simulink library "BLE_Library"  (R2017b)
settings: Solver=VariableStepAuto  StartTime=0.0  StopTime=10.0  RelTol=1e-3
values from neighbouring files (symbols this model uses):
  D = D/ScaleCoefficient    [BLE_PostLoad.m]    (also in new_BLE_model.m = zeros(N_BLE,N_BLE+1))
undefined symbols (not defined in the file or in its folder): ADV_IND_AccA, ADV_IND_id, BT_Hop_Separation, BT_Samples_Per_Symbol, CONNECT_IND_id, CONNECT_IND_length, F3B672D172DF, F506B10B1B3E, Header, LL_DATA_EMPTY_length, LL_DATA_id, magnitude, Payload, Preamble, Slot_Ts, T_IFS
libraries: BLE_Library x56, simulink x39, commutil2 x29, dspindex x17, commdigbbndfm2 x5, dspsigops x2, commrandsrc3 x2, dspstat3 x2, dspsrcs4 x1, dsparch4 x1, commdigbbndcpm2 x1
(part 1 of 5)
settings Model: Creator=rolands  LastModifiedBy=rolands

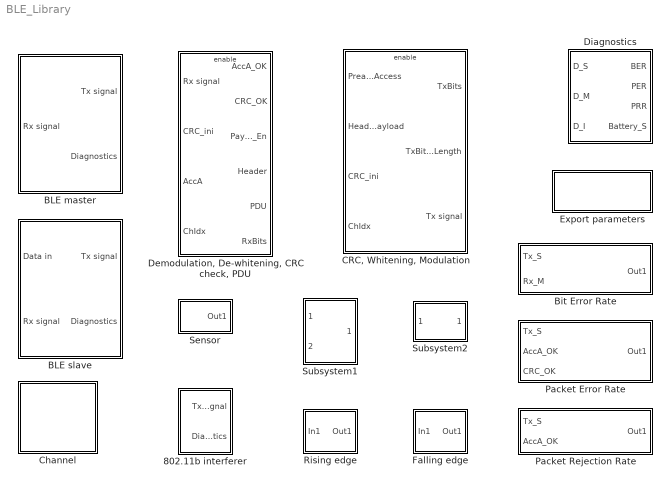
== system BLE_Library ==
  802.11b interferer : Subsystem  mask{rate=70, m=144+48+1024*8 %Preamble + Header + Payload, interference_frequency_number=11}
      mask prompts: rate "Average rate (packets per second):"; m "Mean packet length (us):"; interference_frequency_number "Interference frequency number (1-13, typical: 1, 6 or 11):"
      mask init:
      | interference_frequency_number=min(interference_frequency_number,13);
      | interference_frequency_number=max(interference_frequency_number,1);
      mask Display: disp('802.11b\ninterferer')
  BLE master : Subsystem  StopFcn=|  mask{tON=0, IniState=Initiating, TxAdd=random, InitA_P='112233445566', InitA_R=F506B10B1B3E, PDU_Type=CONNECT_IND, RFU=0, ChSel=0, scanWindow=3500, scanInterval=4500, T_IFS=T_IFS, Interval=6, WinOffset=1, WinSize=1, Timeout=10, Latency=0, SCA=7, DacqSc=MD bit is used (supports only one slave; sampling rate does not exceed 2.136 kHz), NDM=off, DLvalue=off, DataLength=5}
      | uData=get_param(gcb,'UserData');
      | if ~isempty(uData)
      |    if isfield(uData,'AccA_List')
      |       uData=rmfield(uData,'AccA_List');
      |       set_param(gcb,'UserData',uData)
      |    end
      | end
      mask prompts: tON "Turn ON time (us) (>=0 us):"; IniState "Initial state:"; TxAdd "Initiator's address:"; InitA_P "Enter address (hex format, 12 symbols):"; InitA_R "Random address:"; PDU_Type "PDU type:"; scanWindow "Scan window (us) (<=40.96 s):"; scanInterval "Scan interval (us) (<=40.96 s):"; T_IFS "Inter Frame Space (us):"; Interval "Connection Interval (n*1.25 ms, n=6...3200):"; WinOffset "Transmit Window Offset (m*1.25 ms, m=0...n):"; WinSize "Transmit Window Size (k*1.25 ms, k=1...min(8,n-1)):"; Timeout "Connection Supervision Timeout (u*10 ms, u=max(10,floor(n/4)+1)...3200):"; Latency "Connection Slave Latency (0...min(floor(4u/n)-1,499)):"; SCA "Master SCA (0...7):"; NDM "Non-disruptive mode"; DLvalue "Data length is forced to be (1...251 octets):"
      mask init:
      | tON=max(round(tON),0); %minimum value 0 us
      | 
      | scanInterval=min(scanInterval,40.96e6);
      | scanWindow=min(scanWindow,scanInterval);
      | 
      | Interval=max(Interval,6);
      | Interval=min(Interval,3200);
      | 
      | Nsl=ceil(Interval*1250/2500); %max number of slaves in multiple slaves mode
      | 
      | WinOffset=min(WinOffset,Interval);
      | 
      | WinSize=max(WinSize,1);
      | WinSize=min(WinSize,min(8,Interval-1));
      | 
      | Timeout=max(Timeout,max(10,floor(Interval/4)+1));
      | Timeout=min(Timeout,3200);
      | 
      | Latency=max(Latency,0);
      | Latency=min(Latency,min(floor(4*Timeout/Interval)-1,499));
      | 
      | SCA=max(SCA,0);
      | SCA=min(SCA,7);
      | 
      | 
      | switch get_param(gcb,'DacqSc')    %master mode
      |     case 'MD bit is used (supports only one slave; sampling rate does not exceed 2.136 kHz)'        
      |         set_param([gcb,'/Master mode'],'OverrideUsingVariant','OneSlaveMode')     
      |     otherwise
      |         set_param([gcb,'/Master mode'],'OverrideUsingVariant','MultipleSlavesMode')
      | end
      | 
      | 
      | name=get_param(gcb,'name');
      | if name(5)=='m'
      |     nD=name(11:length(name)); %device number
      | elseif name(5)=='s'
      |     nD=name(10:length(name));
      | else
      |     nD='x';
      | end
      | nD=double(nD);
      | 
      | 
      | if strcmp(get_param(gcb,'TxAdd'),'public')
      |     u2=get_param(gcb,'InitA_P');
      |     InitA=dec2bin(hex2dec(u2(2:end-1)),48);
      | else
      |     u2=get_param(gcb,'InitA_R');
      |     InitA=dec2bin(hex2dec(u2),48);
      | end
      | InitA=reshape(InitA.',1,[])-'0';
      | InitA=InitA';
      | 
      | 
      | 
      | slave_AdvAs=zeros(48,8);
      | slave_Names=zeros(1,8);
      | 
      | Names=find_system(bdroot,'regexp','on','Name','BLE slave');
      | if ~isempty(Names)
      |     for k=1:length(Names)
      |         slave_AdvAs(:,k)=getfield(get_param(Names{k},'UserData'),'bin');
      |         name=get_param(Names{k},'Name');
      |         slave_Names(k)=str2num(name(10:end));
      |     end
      | end
      settings: CopyFcn=|
      | if isempty(who('AdvA_List'))
      |    AdvA_List=[];
      | else
      |    AdvA_List=evalin('base','AdvA_List');
      | end
      | 
      | [RandA_bin,RandA_hex, AdvA_List] = GenStatDevAddr(AdvA_List);
      | set_param(gcb,'UserData',struct('bin',RandA_bin,'hex',RandA_hex));
      | set_param(gcb,'InitA_R',RandA_hex);
      settings: DeleteFcn=|
      | if ~isempty(who('AdvA_List'))
      |    AdvA_List=evalin('base','AdvA_List');
      |    add=get_param(gcb,'UserData');
      |    if ~isempty(add)
      |       for k=1:size(AdvA_List,1)
      |          if strcmp(add.hex,AdvA_List(k,:))
      |             AdvA_List(k,:)=[];
      |             break;
      |          end
      |       end
      |    end
      | end
      settings: UndoDeleteFcn=|
      | if isempty(who('AdvA_List'))
      |    AdvA_List=[];
      | else
      |    AdvA_List=evalin('base','AdvA_List');
      | end
      | 
      | add=get_param(gcb,'UserData');
      | if ~isempty(add)
      |    AdvA_List=[AdvA_List; add.hex];
      |    set_param(gcb,'InitA_R',add.hex);
      | else
      |    [RandA_bin,RandA_hex, AdvA_List] = GenStatDevAddr(AdvA_List);
      |    set_param(gcb,'UserData',struct('bin',RandA_bin,'hex',RandA_hex));
      |    set_param(gcb,'InitA_R',RandA_hex);
      | end
      mask TypeOptions IniState: Initiating
      mask TypeOptions TxAdd: public | random
      mask Callback TxAdd:
      | Names = get_param(gcb,'MaskNames');
      | NamesVis = get_param(gcb,'MaskVisibilities');
      | NamesEn = get_param(gcb,'MaskEnables');
      | NameIdx1 = find(strcmp(Names,'InitA_P'));
      | NameIdx2 = find(strcmp(Names,'InitA_R'));
      | 
      | if strcmp(get_param(gcb,'TxAdd'),'public')
      |     NamesVis{NameIdx1}='on';
      |     NamesVis{NameIdx2}='off';
      |     set_param(gcb,'MaskVisibilities',NamesVis);
      | else
      |     NamesVis{NameIdx1}='off';
      |     NamesVis{NameIdx2}='on';
      |     NamesEn{NameIdx2}='off';
      |     set_param(gcb,'MaskVisibilities',NamesVis);
      |     AdvA_List=evalin('base','AdvA_List');
      |     add=get_param(gcb,'UserData');
      |     if isempty(add)
      |         [RandA_bin,RandA_hex, AdvA_List] = GenStatDevAddr(AdvA_List);
      |         assignin('base','AdvA_List',AdvA_List)
      |         add.bin=RandA_bin;
      |         add.hex=RandA_hex;
      |         set_param(gcb,'UserData',add);
      |     else
      |         flag=0;
      |         for k=1:size(AdvA_List,1)
      |             if strcmp(add.hex,AdvA_List(k,:))
      |                 flag=1;
      |                 break;
      |             end
      |         end
      |         if flag~=1
      |             assignin('base','AdvA_List',[AdvA_List;add.hex]);
      |         end
      |     end
      |     set_param(gcb,'InitA_R',add.hex);
      |     set_param(gcb,'MaskEnables',NamesEn);
      | end
      mask TypeOptions PDU_Type: CONNECT_IND
      mask TypeOptions RFU: 0 | 1
      mask TypeOptions ChSel: 0 | 1
      mask TypeOptions DacqSc: MD bit is used (supports only one slave; sampling rate does not exceed 2.136 kHz) | MD bit is ignored (supports multiple slaves; sampling rates do not exceed 0.133 kHz)
      mask Callback DacqSc:
      | Names = get_param(gcb,'MaskNames');
      | NamesVis = get_param(gcb,'MaskVisibilities');
      | NameIdx = find(strcmp(Names,'NDM'));
      | NameIdx1 = find(strcmp(Names,'DLvalue'));
      | NameIdx2 = find(strcmp(Names,'DataLength'));
      | 
      | if strcmp(get_param(gcb,'DacqSc'),'MD bit is used (supports only one slave; sampling rate does not exceed 2.136 kHz)')
      |     NamesVis{NameIdx}='on';
      |     NamesVis{NameIdx1}='on';
      |     NamesVis{NameIdx2}='on';
      |     set_param([gcb,'/Master mode'],'OverrideUsingVariant','OneSlaveMode')
      | else
      |     NamesVis{NameIdx}='off';
      |     NamesVis{NameIdx1}='off';
      |     NamesVis{NameIdx2}='off';
      |     set_param([gcb,'/Master mode'],'OverrideUsingVariant','MultipleSlavesMode')
      | end
      | 
      | set_param(gcb,'MaskVisibilities',NamesVis)
      mask Callback DLvalue:
      | Names = get_param(gcb,'MaskNames');
      | NamesEn = get_param(gcb,'MaskEnables');
      | NameIdx = find(strcmp(Names,'DataLength'));
      | 
      | if strcmp(get_param(gcb,'DLvalue'),'on')
      |     NamesEn{NameIdx}='on';
      | else
      |     NamesEn{NameIdx}='off';
      | end
      | 
      | set_param(gcb,'MaskEnables',NamesEn)
      mask DialogControl Container6 Prompt: Data acquisition mode
      mask Display:
      | if strcmp(get_param(gcb,'TxAdd'),'public')
      |     add=get_param(gcb,'InitA_P');
      |     disp(['PA: ',add(2:end-1),'\n\n\n\n\n\n\n\n\n\n\n\n'])
      | else
      |     disp(['RA: ',get_param(gcb,'InitA_R'),'\n\n\n\n\n\n\n\n\n\n\n\n'])
      | end
      | plot(0,0,100,100,[35,65,65,60,60,35,35],[10,10,90,90,75,75,10],[40,40,60,60,40],[69,50,50,69,69],[48,55,55,50,50,55,55,48],[18,25,25,30,30,35,35,42],[48,43,48,43,43,44,44,48],[30,35,30,25,25,24,24,28],[48,48],[32,42],[48,48],[18,28],[43,44,44,48],[35,36,36,32],[53,49.5,49.5,49.5,49.5,53],[25,28.5,28.5,21.5,21.5,25],[53,49.5,49.5,49.5,49.5,53],[35,38.5,38.5,31.5,31.5,35])
  BLE slave : Subsystem  mask{tON=1, IniState=Advertising, TxAdd=random, AdvA_P='778899AABBCC', AdvA_R=F3B672D172DF, PDU_Type=ADV_IND, RFU=0, ChSel=0, RxAdd=random, TargA_PR=C4CA1158607C, T_ADV_IND_in=1, advInterval_in=20, MDbit=on, NDM=off, SamplParam=2,000 kHz (500 us), 5, 15, 7.5 ms, Fs=1000/500, n_data=5, m_packets=15, Interval_ms=6, BatU=3.6, BatC=2400, Idle_Power=10, Energy_per_sbit=10, Energy_per_rbit=2, BatChargPower=0}
      mask prompts: tON "Turn ON time: (us) (>=1 us)"; IniState "Initial state:"; TxAdd "Advertiser's address:"; AdvA_P "Enter address (hex format, 12 symbols):"; AdvA_R "Random address:"; PDU_Type "PDU type:"; RxAdd "Target's address:"; TargA_PR "Choose from the list:"; T_ADV_IND_in "Time between two consecutive ADV_IND PDUs (ms) (<=10 ms):"; advInterval_in "advInterval (ms) [20 ms ... 10485759.375ms]:"; MDbit "MD bit is used"; NDM "Non-disruptive mode"; SamplParam "Choose from the following:"; Fs "Sampling frequency (kHz):"; n_data "Data length (1 ... 251 octets):"; m_packets "Data packets per connection interval:"; Interval_ms "Required connection interval (n*1.25 ms, n=6...3200):"; BatU "Voltage (V):"; BatC "Capacity (mAh):"; Idle_Power "Idle state power consumption (uW):"; Energy_per_sbit "Energy spent per bit sent (uJ):"; Energy_per_rbit "Energy spent per bit received (uJ):"; BatChargPower "Battery charging power (W):"
      mask init:
      | tON=max(round(tON),1); %minimum value 1 us
      | 
      | T_ADV_IND=round(T_ADV_IND_in*1000); %us
      | T_ADV_IND=min(T_ADV_IND,10000); %maximum value 10 ms
      | 
      | advInterval=round(advInterval_in/0.625)*0.625; %ms
      | advInterval=max(advInterval,20); %minimum value 20 ms 
      | advInterval=min(advInterval,10485759.375); %maximum value 10485759.375 ms
      | advInterval=advInterval*1000; %us
      | 
      | advInterval=max(T_ADV_IND*3,advInterval);
      | 
      | name=get_param(gcb,'name');
      | if name(5)=='m'
      |     nD=name(11:length(name)); %device number
      | elseif name(5)=='s'
      |     nD=name(10:length(name));
      | else
      |     nD='x';
      | end
      | nD=double(nD);
      | 
      | 
      | if strcmp(get_param(gcb,'TxAdd'),'public')
      |     u2=get_param(gcb,'AdvA_P');
      |     AdvA=dec2bin(hex2dec(u2(2:end-1)),48);
      | else
      |     u2=get_param(gcb,'AdvA_R');
      |     AdvA=dec2bin(hex2dec(u2),48);
      | end
      | AdvA=reshape(AdvA.',1,[])-'0';
      | AdvA=AdvA';
      | 
      | u2=get_param(gcb,'TargA_PR');
      | TargA=dec2bin(hex2dec(u2),48);
      | TargA=reshape(TargA.',1,[])-'0';
      | TargA=TargA';
      | 
      | 
      | 
      | master_AdvAs=zeros(48,8);
      | master_Names=zeros(8,1);
      | 
      | Names=find_system(bdroot,'regexp','on','Name','BLE master');
      | if ~isempty(Names)
      |     for k=1:length(Names)
      |         master_AdvAs(:,k)=getfield(get_param(Names{k},'UserData'),'bin');
      |         name=get_param(Names{k},'Name');
      |         master_Names(k)=str2num(name(11:end));
      |     end
      | end
      settings: CopyFcn=|
      | if isempty(who('AdvA_List'))
      |    AdvA_List=[];
      | else
      |    AdvA_List=evalin('base','AdvA_List');
      | end
      | 
      | [RandA_bin,RandA_hex, AdvA_List] = GenStatDevAddr(AdvA_List);
      | set_param(gcb,'UserData',struct('bin',RandA_bin,'hex',RandA_hex));
      | set_param(gcb,'AdvA_R',RandA_hex);
      settings: DeleteFcn=|
      | if ~isempty(who('AdvA_List'))
      |    AdvA_List=evalin('base','AdvA_List');
      |    add=get_param(gcb,'UserData');
      |    if ~isempty(add)
      |       for k=1:size(AdvA_List,1)
      |          if strcmp(add.hex,AdvA_List(k,:))
      |             AdvA_List(k,:)=[];
      |             break;
      |          end
      |       end
      |    end
      | end
      settings: UndoDeleteFcn=|
      | if isempty(who('AdvA_List'))
      |    AdvA_List=[];
      | else
      |    AdvA_List=evalin('base','AdvA_List');
      | end
      | 
      | add=get_param(gcb,'UserData');
      | if ~isempty(add)
      |    AdvA_List=[AdvA_List; add.hex];
      |    set_param(gcb,'AdvA_R',add.hex);
      | else
      |    [RandA_bin,RandA_hex, AdvA_List] = GenStatDevAddr(AdvA_List);
      |    set_param(gcb,'UserData',struct('bin',RandA_bin,'hex',RandA_hex));
      |    set_param(gcb,'AdvA_R',RandA_hex);
      | end
      mask TypeOptions IniState: Advertising
      mask TypeOptions TxAdd: public | random
      mask Callback TxAdd:
      | NamesM = get_param(gcb,'MaskNames');
      | NamesVisM = get_param(gcb,'MaskVisibilities');
      | NamesEnM = get_param(gcb,'MaskEnables');
      | NameMIdx1 = find(strcmp(NamesM,'AdvA_P'));
      | NameMIdx2 = find(strcmp(NamesM,'AdvA_R'));
      | 
      | if strcmp(get_param(gcb,'TxAdd'),'public')
      |     NamesVisM{NameMIdx1}='on';
      |     NamesVisM{NameMIdx2}='off';
      |     set_param(gcb,'MaskVisibilities',NamesVisM);
      | else
      |     NamesVisM{NameMIdx1}='off';
      |     NamesVisM{NameMIdx2}='on';
      |     NamesEnM{NameMIdx2}='off';
      |     set_param(gcb,'MaskVisibilities',NamesVisM);
      |     AdvA_List=evalin('base','AdvA_List');
      |     add=get_param(gcb,'UserData');
      |     if isempty(add)
      |         [RandA_bin,RandA_hex, AdvA_List] = GenStatDevAddr(AdvA_List);
      |         assignin('base','AdvA_List',AdvA_List)
      |         add.bin=RandA_bin;
      |         add.hex=RandA_hex;
      |         set_param(gcb,'UserData',add);
      |     else
      |         flag=0;
      |         for k=1:size(AdvA_List,1)
      |             if strcmp(add.hex,AdvA_List(k,:))
      |                 flag=1;
      |                 break;
      |             end
      |         end
      |         if flag~=1
      |             assignin('base','AdvA_List',[AdvA_List;add.hex]);
      |         end
      |     end
      |     set_param(gcb,'AdvA_R',add.hex);
      |     set_param(gcb,'MaskEnables',NamesEnM);
      | end
      mask TypeOptions PDU_Type: ADV_IND | ADV_DIRECT_IND
      mask Callback PDU_Type:
      | NamesS = get_param(gcb,'MaskNames');
      | NamesVisS = get_param(gcb,'MaskVisibilities');
      | NameSIdx1 = find(strcmp(NamesS,'RxAdd'));
      | NameSIdx2 = find(strcmp(NamesS,'TargA_PR'));
      | hmask=Simulink.Mask.get(gcb);
      | 
      | if strcmp(get_param(gcb,'PDU_Type'),'ADV_IND')
      |     NamesVisS{NameSIdx1}='off';
      |     NamesVisS{NameSIdx2}='off';
      |     hmask.getDialogControl('ConfigureM').Visible='off';
      |     set_param(gcb,'MaskVisibilities',NamesVisS);
      | else
      |     m_Add=[]; kk=1;
      |     Names=find_system(bdroot,'regexp','on','Name','BLE master');
      |     if ~isempty(Names)
      |         for k=1:length(Names)
      |             if strcmp(get_param(Names{k},'TxAdd'),'random')
      |                 addr=get_param(Names{k},'InitA_R');
      |             else
      |                 addr=get_param(Names{k},'InitA_P');
      |                 addr=addr(2:end-1);
      |             end
      |             m_Add=[m_Add; {addr}];
      |             if strcmp(hmask.Parameters(10).Value, addr)
      |                 kk=k;
      |             end
      |         end
      |         hmask.Parameters(10).set('TypeOptions',m_Add,'Value',m_Add{kk});
      |     end
      |     NamesVisS{NameSIdx1}='on';
      |     NamesVisS{NameSIdx2}='on';
      |     hmask.getDialogControl('ConfigureM').Visible='on';
      |     set_param(gcb,'MaskVisibilities',NamesVisS);
      |     set_param(gcb,'RxAdd',get_param(Names{kk},'TxAdd'));
      | end
      mask TypeOptions RFU: 0 | 1
      mask TypeOptions ChSel: 0 | 1
      mask TypeOptions RxAdd: public | random
      mask TypeOptions TargA_PR: C4CA1158607C
      mask Callback TargA_PR:
      | if strcmp(get_param(gcb,'PDU_Type'),'ADV_DIRECT_IND')
      | 
      |     name=get_param(gcb,'TargA_PR');
      |     Names=find_system(bdroot,'regexp','on','Name','BLE master');
      |     if ~isempty(Names)
      |         for k=1:length(Names)
      | 
      |             if strcmp(get_param(Names{k},'TxAdd'),'random')
      |                 initA=get_param(Names{k},'InitA_R');
      |             else
      |                 addr=get_param(Names{k},'InitA_P');
      |                 initA=addr(2:end-1);
      |             end
      | 
      |             if strcmp(name,initA)
      |                 set_param(gcb,'RxAdd',get_param(Names{k},'TxAdd'));
      |                 break;
      |             end
      |         end
      |     end
      | end
      mask Callback MDbit:
      | NamesS = get_param(gcb,'MaskNames');
      | NamesVisS = get_param(gcb,'MaskVisibilities');
      | NamesEnS = get_param(gcb,'MaskEnables');
      | NameSIdx = find(strcmp(NamesS,'NDM'));
      | NameSIdx1 = find(strcmp(NamesS,'SamplParam'));
      | NameSIdx2 = find(strcmp(NamesS,'n_data'));
      | NameSIdx3 = find(strcmp(NamesS,'Interval_ms'));
      | 
      | if strcmp(get_param(gcb,'MDbit'),'on')
      |     NamesVisS{NameSIdx}='on';
      |     NamesVisS{NameSIdx1}='on';
      |     NamesEnS{NameSIdx2}='off';
      |     NamesEnS{NameSIdx3}='off';
      | else
      |     NamesVisS{NameSIdx}='off';
      |     NamesVisS{NameSIdx1}='off';
      |     NamesEnS{NameSIdx2}='on';
      |     NamesEnS{NameSIdx3}='on';
      | end
      | set_param(gcb,'MaskVisibilities',NamesVisS)
      | set_param(gcb,'MaskEnables',NamesEnS)
      | 
      | 
      | if strcmp(get_param(gcb,'MDbit'),'on')
      |     if strcmp(get_param(gcb,'SamplParam'),'2.137 kHz (468 us), 1, 625, 292.5 ms')
      |         set_param(gcb,'Fs','1000/468','n_data','1','m_packets','625','Interval_ms','234');
      |     elseif strcmp(get_param(gcb,'SamplParam'),'2.066 kHz (484 us), 3, 625, 302.5 ms')
      |         set_param(gcb,'Fs','1000/484','n_data','3','m_packets','625','Interval_ms','242');
      |     elseif strcmp(get_param(gcb,'SamplParam'),'2,000 kHz (500 us), 5, 15, 7.5 ms')
      |         set_param(gcb,'Fs','1000/500','n_data','5','m_packets','15','Interval_ms','6');
      |     elseif strcmp(get_param(gcb,'SamplParam'),'1.852 kHz (540 us), 10, 125, 67.5 ms')
      |         set_param(gcb,'Fs','1000/540','n_data','10','m_packets','125','Interval_ms','54');
      |     elseif strcmp(get_param(gcb,'SamplParam'),'1.724 kHz (580 us), 15, 125, 72.5 ms')
      |         set_param(gcb,'Fs','1000/580','n_data','15','m_packets','125','Interval_ms','58');
      |     elseif strcmp(get_param(gcb,'SamplParam'),'1.613 kHz (620 us), 20, 125, 77.5 ms')
      |         set_param(gcb,'Fs','1000/620','n_data','20','m_packets','125','Interval_ms','62');
      |     elseif strcmp(get_param(gcb,'SamplParam'),'1.515 kHz (660 us), 25, 125, 82.5 ms')
      |         set_param(gcb,'Fs','1000/660','n_data','25','m_packets','125','Interval_ms','66');
      |     elseif strcmp(get_param(gcb,'SamplParam'),'1.429 kHz (700 us), 30, 25, 17.5 ms')
      |         set_param(gcb,'Fs','1000/700','n_data','30','m_packets','25','Interval_ms','14');
      |     elseif strcmp(get_param(gcb,'SamplParam'),'1.111 kHz (900 us), 55, 25, 22.5 ms')
      |         set_param(gcb,'Fs','1000/900','n_data','55','m_packets','25','Interval_ms','18');
      |     elseif strcmp(get_param(gcb,'SamplParam'),'0.667 kHz (1500 us), 130, 5, 7.5 ms')
      |         set_param(gcb,'Fs','1000/1500','n_data','130','m_packets','5','Interval_ms','6');
      |     elseif strcmp(get_param(gcb,'SamplParam'),'0.435 kHz (2300 us), 230, 25, 57.5 ms')
      |         set_param(gcb,'Fs','1000/2300','n_data','230','m_packets','25','Interval_ms','46');
      |     else
      |         set_param(gcb,'Fs','1000/7500','n_data','1','m_packets','5','Interval_ms','6');
      |     end
      | else
      |     set_param(gcb,'Fs',['0.8/',get_param(gcb,'Interval_ms'),' (denominator follows from the connection interval)'],'m_packets','1');
      | end
      mask TypeOptions SamplParam: 2.137 kHz (468 us), 1, 625, 292.5 ms | 2.066 kHz (484 us), 3, 625, 302.5 ms | 2,000 kHz (500 us), 5, 15, 7.5 ms | 1.852 kHz (540 us), 10, 125, 67.5 ms | 1.724 kHz (580 us), 15, 125, 72.5 ms | 1.613 kHz (620 us), 20, 125, 77.5 ms | 1.515 kHz (660 us), 25, 125, 82.5 ms | 1.429 kHz (700 us), 30, 25, 17.5 ms | 1.111 kHz (900 us), 55, 25, 22.5 ms | 0.667 kHz (1500 us), 130, 5, 7.5 ms | 0.435 kHz (2300 us), 230, 25, 57.5 ms | 0.133 kHz (7500 us), 1, 5, 7.5 ms (non-uniform)
      mask Callback SamplParam:
      | if strcmp(get_param(gcb,'MDbit'),'on')
      |     if strcmp(get_param(gcb,'SamplParam'),'2.137 kHz (468 us), 1, 625, 292.5 ms')
      |         set_param(gcb,'Fs','1000/468','n_data','1','m_packets','625','Interval_ms','234');
      |     elseif strcmp(get_param(gcb,'SamplParam'),'2.066 kHz (484 us), 3, 625, 302.5 ms')
      |         set_param(gcb,'Fs','1000/484','n_data','3','m_packets','625','Interval_ms','242');
      |     elseif strcmp(get_param(gcb,'SamplParam'),'2,000 kHz (500 us), 5, 15, 7.5 ms')
      |         set_param(gcb,'Fs','1000/500','n_data','5','m_packets','15','Interval_ms','6');
      |     elseif strcmp(get_param(gcb,'SamplParam'),'1.852 kHz (540 us), 10, 125, 67.5 ms')
      |         set_param(gcb,'Fs','1000/540','n_data','10','m_packets','125','Interval_ms','54');
      |     elseif strcmp(get_param(gcb,'SamplParam'),'1.724 kHz (580 us), 15, 125, 72.5 ms')
      |         set_param(gcb,'Fs','1000/580','n_data','15','m_packets','125','Interval_ms','58');
      |     elseif strcmp(get_param(gcb,'SamplParam'),'1.613 kHz (620 us), 20, 125, 77.5 ms')
      |         set_param(gcb,'Fs','1000/620','n_data','20','m_packets','125','Interval_ms','62');
      |     elseif strcmp(get_param(gcb,'SamplParam'),'1.515 kHz (660 us), 25, 125, 82.5 ms')
      |         set_param(gcb,'Fs','1000/660','n_data','25','m_packets','125','Interval_ms','66');
      |     elseif strcmp(get_param(gcb,'SamplParam'),'1.429 kHz (700 us), 30, 25, 17.5 ms')
      |         set_param(gcb,'Fs','1000/700','n_data','30','m_packets','25','Interval_ms','14');
      |     elseif strcmp(get_param(gcb,'SamplParam'),'1.111 kHz (900 us), 55, 25, 22.5 ms')
      |         set_param(gcb,'Fs','1000/900','n_data','55','m_packets','25','Interval_ms','18');
      |     elseif strcmp(get_param(gcb,'SamplParam'),'0.667 kHz (1500 us), 130, 5, 7.5 ms')
      |         set_param(gcb,'Fs','1000/1500','n_data','130','m_packets','5','Interval_ms','6');
      |     elseif strcmp(get_param(gcb,'SamplParam'),'0.435 kHz (2300 us), 230, 25, 57.5 ms')
      |         set_param(gcb,'Fs','1000/2300','n_data','230','m_packets','25','Interval_ms','46');
      |     else
      |         set_param(gcb,'Fs','1000/7500','n_data','1','m_packets','5','Interval_ms','6');
      |     end
      | end
      mask Callback Interval_ms:
      | if strcmp(get_param(gcb,'MDbit'),'off')
      |     set_param(gcb,'Fs',['0.8/',get_param(gcb,'Interval_ms'),' (denominator follows from the connection interval)']);
      | end
      mask DialogControl Container3 Prompt: Sampling parameters
      mask DialogControl ConfigureM Prompt: Configure the master device accordingly
      mask DialogControl ConfigureM Callback:
      | if strcmp(get_param(gcb,'PDU_Type'),'ADV_DIRECT_IND')
      | 
      |     name=get_param(gcb,'TargA_PR');
      |     Names=find_system(bdroot,'regexp','on','Name','BLE master');
      |     if ~isempty(Names)
      |         for k=1:length(Names)
      | 
      |             if strcmp(get_param(Names{k},'TxAdd'),'random')
      |                 initA=get_param(Names{k},'InitA_R');
      |             else
      |                 addr=get_param(Names{k},'InitA_P');
      |                 initA=addr(2:end-1);
      |             end
      | 
      |             if strcmp(name,initA)
      |                 set_param(Names{k},'Interval',get_param(gcb,'Interval_ms'));
      | 
      |                 NamesM = get_param(Names{k},'MaskNames');
      |                 NamesVisM = get_param(Names{k},'MaskVisibilities');
      |                 NameMIdx1 = find(strcmp(NamesM,'NDM'));
      |                 NameMIdx2 = find(strcmp(NamesM,'DLvalue'));
      |                 NameMIdx3 = find(strcmp(NamesM,'DataLength'));
      | 
      |                 if strcmp(get_param(gcb,'MDbit'),'on')
      |                     set_param(Names{k},'DacqSc','MD bit is used (supports only one slave; sampling rate does not exceed 2.136 kHz)')
      |                     set_param([Names{k},'/Master mode'],'OverrideUsingVariant','OneSlaveMode')
      |                     ndm=get_param(gcb,'NDM');
      |                     NamesVisM{NameMIdx1}='on';
      |                     NamesVisM{NameMIdx2}='on';
      |                     NamesVisM{NameMIdx3}='on';
      |                 else
      |                     set_param(Names{k},'DacqSc','MD bit is ignored (supports multiple slaves; sampling rates do not exceed 0.133 kHz)')
      |                     set_param([Names{k},'/Master mode'],'OverrideUsingVariant','MultipleSlavesMode')
      |                     ndm='off';
      |                     NamesVisM{NameMIdx1}='off';
      |                     NamesVisM{NameMIdx2}='off';
      |                     NamesVisM{NameMIdx3}='off';
      |                 end
      | 
      |                 set_param(Names{k},'MaskVisibilities',NamesVisM)
      |                 set_param(Names{k},'NDM',ndm)
      |                 set_param(Names{k},'DataLength',get_param(gcb,'n_data'))
      |                 break;
      |             end
      |         end
      |     end
      | end
      mask DialogControl Container6 Prompt: Battery parameters
      mask Display:
      | if strcmp(get_param(gcb,'TxAdd'),'public')
      |     add=get_param(gcb,'AdvA_P');
      |     disp(['PA: ',add(2:end-1),'\n\n\n\n\n\n\n\n\n\n\n\n'])
      | else
      |     disp(['RA: ',get_param(gcb,'AdvA_R'),'\n\n\n\n\n\n\n\n\n\n\n\n'])
      | end
      | 
      | if strcmp(get_param(gcb,'PDU_Type'),'ADV_DIRECT_IND')
      |     add=get_param(gcb,'TargA_PR');
      |     if strcmp(get_param(gcb,'RxAdd'),'public')
      |         disp(['\n\n\n\n\n\n\n\n\n\n\n\n','TA: ',add(2:end-1)])
      |     else
      |         disp(['\n\n\n\n\n\n\n\n\n\n\n\n','TA: ',add])
      |     end
      | end
      | 
      | plot(0,0,100,100,[35,65,65,60,60,35,35],[10,10,90,90,75,75,10],[40,40,60,60,40],[69,50,50,69,69],[48,55,55,50,50,55,55,48],[18,25,25,30,30,35,35,42],[48,43,48,43,43,44,44,48],[30,35,30,25,25,24,24,28],[48,48],[32,42],[48,48],[18,28],[43,44,44,48],[35,36,36,32],[53,49.5,49.5,49.5,49.5,53],[25,28.5,28.5,21.5,21.5,25],[53,49.5,49.5,49.5,49.5,53],[35,38.5,38.5,31.5,31.5,35])
  Bit Error Rate : Subsystem
      mask Display: disp('BER\n calculation')
  "CRC, Whitening, Modulation" : Subsystem
  Channel : Subsystem  InitFcn=|  mask{Tx_power=0, Channel_SNR=-20, InterfOn=off, Interf_power=10}
      | XY=[];
      | Names=find_system(bdroot,'regexp','on','Name','BLE master');
      | if ~isempty(Names)
      |     for k=1:length(Names)
      |         xy=get_param(Names{k},'Position');
      |         XY=[XY;xy(1:2)];
      |     end
      | end
      | 
      | Names=find_system(bdroot,'regexp','on','Name','BLE slave');
      | if ~isempty(Names)
      |     for k=1:length(Names)
      |         xy=get_param(Names{k},'Position');
      |         XY=[XY;xy(1:2)];
      |     end
      | end
      | 
      | Names=find_system(bdroot,'regexp','on','Name','interferer');
      | if ~isempty(Names)
      |     for k=1:length(Names)
      |         xy=get_param(Names{k},'Position');
      |         XY=[XY;xy(1:2)];
      |     end
      | end
      | 
      | if ~isempty(XY)
      |     N_BLE=size(XY,1)-1;
      |     D=zeros(N_BLE,N_BLE+1);
      |     for n=1:size(XY,1)
      |         for k=1:size(XY,1)
      |             D(n,k)=sqrt((XY(n,1)-XY(k,1))^2+(XY(n,2)-XY(k,2))^2);
      |         end
      |     end
      |     ScaleCoefficient=0;
      |     varList=whos(get_param(bdroot,'ModelWorkspace'));
      |     if ~isempty(varList)
      |         for m=1:length(varList)
      |             if strcmp(varList(m).name,'ScaleCoefficient')
      |                 ScaleCoefficient=getVariable(get_param(bdroot,'ModelWorkspace'),'ScaleCoefficient');
      |                 break;
      |             end
      |         end
      |     end
      |     if ScaleCoefficient==0
      |         ScaleCoefficient=1;
      |     end
      |     D=D/ScaleCoefficient;
      |     
      |     D_path_loss=1./(4*pi*D*2.4e9/299792458);
      |     D_path_loss(D_path_loss==Inf)=0;
      |     assignin('base', 'D', D');
      |     assignin('base', 'D_path_loss_I_on', D_path_loss');
      |     D_path_loss(:,end)=0;
      |     assignin('base', 'D_path_loss_I_off', D_path_loss');
      | end
      mask prompts: Tx_power "BLE transmit power (-20 dBm ... +10 dBm):"; Channel_SNR "AWGN channel noise power (dBm):"; InterfOn "Interferer On"; Interf_power "Interferer transmit power (<= +20 dBm):"
  "Demodulation, De-whitening, CRC check, PDU" : Subsystem  mask{PDU_Length=112 %ADV_DIRECT_IND: 2+6+6 octets (H,AdvA,TargetA), N_after=136 %max PDU length + CRC}
      mask prompts: PDU_Length "PDU length (number of bits):"; N_after "Counter limit after AccA OK:"
  Diagnostics : Subsystem
  Export parameters : Subsystem
      settings: OpenFcn=|
      | if ~exist('Parameters','dir')
      |     mkdir('Parameters')
      | end
      | 
      | set_param(gcb,'BackgroundColor','red')
      | set_param(gcb,'MaskDisplay',"disp('Generating\n.txt file')")
      | pause(0.5)
      | 
      | Names=find_system(bdroot,'regexp','on','Name','BLE master');
      | if ~isempty(Names)
      |     for k=1:length(Names)
      |        ParamNames=get_param(Names{k},'MaskPrompts');
      |        ParamValues=get_param(Names{k},'MaskValues');
      |        writetable(table(ParamNames, ParamValues, 'VariableNames',{'Parameter','Value'}), ['Parameters/Parameters_',get_param(Names{k},'Name'),'.txt'])
      |     end
      | end
      | 
      | Names=find_system(bdroot,'regexp','on','Name','BLE slave');
      | if ~isempty(Names)
      |     for k=1:length(Names)
      |        ParamNames=get_param(Names{k},'MaskPrompts');
      |        ParamValues=get_param(Names{k},'MaskValues');
      |        writetable(table(ParamNames, ParamValues, 'VariableNames',{'Parameter','Value'}), ['Parameters/Parameters_',get_param(Names{k},'Name'),'.txt'])
      |     end
      | end
      | 
      | set_param(gcb,'BackgroundColor','green')
      | set_param(gcb,'MaskDisplay',"disp('Double-click\nto generate\nparameters .txt files')")
      mask Display: disp('Double-click\nto generate\nparameters .txt files')
  Falling edge : Subsystem
      mask Display: disp('Falling\nedge\npulse')
  Packet Error Rate : Subsystem
      mask Display: disp('PER\n calculation')
  Packet Rejection Rate : Subsystem
      mask Display: disp('PRR\n calculation')
  Rising edge : Subsystem
      mask Display: disp('Rising\nedge\npulse')
  Sensor : Subsystem  mask{NbitsPerSample=4}
      mask prompts: NbitsPerSample "Number of bits per sample:"
      mask Display: disp('Sensor')
  Subsystem1 : Subsystem  mask{PDU_type=CONNECT_IND_id}
      mask prompts: PDU_type "PDU type:"
  Subsystem2 : Subsystem  mask{offset=1}
      mask Display: disp('Count\npulses')

== system BLE_Library/802.11b interferer ==
  22MHz white noise : dspsrcs4/Random Source  SrcType=Gaussian  NormMethod=Ziggurat  CltLength=12  MinVal=0  MaxVal=1  MeanVal=0  VarVal=1  RepMode=Not repeatable  rawSeed=awgn_seed  IsInherit=off  SampMode=Discrete  SampTime=Slot_Ts/22  SampFrame=22  DataType=Double  OutComplex=Complex  OutputFrames=off
  Bus Creator : BusCreator  Inputs=2
  Constant1 : Constant  SampleTime=Slot_Ts
  Constant5 : Constant  Value=interference_frequency_number  SampleTime=Slot_Ts
  Digital Filter Design : dsparch4/Digital Filter Design  mwdsp_browser_bugfix_var=off
  Enabled Subsystem : Subsystem  TreatAsAtomicUnit=on
  Gain : Gain  Gain=sqrt(4)  SaturateOnIntegerOverflow=on  OutDataTypeStr=Inherit: Same as input  ParamDataTypeStr=Inherit: Same as input
  Gain1 : Gain  Gain=2.7  SaturateOnIntegerOverflow=on  OutDataTypeStr=Inherit: Same as input  ParamDataTypeStr=Inherit: Same as input
  M-FSK Modulator Baseband : commdigbbndfm2/M-FSK Modulator Baseband  M=13  InType=Integer  Enc=Binary  freqSep=5e6  phaseType=Continuous  numSamp=BT_Samples_Per_Symbol  RateOptions=Enforce single-rate processing  outDataType=double
      settings: SourceProductName=Communications System Toolbox
  Mix to appropriate hop frequency : Product  SaturateOnIntegerOverflow=on  InputSameDT=on  OutDataTypeStr=Inherit: Same as first input
  Poisson pulses : Subsystem  mask{average_rate=rate, packet_length=m*Slot_Ts}
      mask prompts: average_rate "Average rate (packets per second):"; packet_length "Mean packet length:"
      mask init:
      | adjusted_rate=1/(1/average_rate-packet_length);
  Sum : Sum  Inputs=|+-
  Upsample to 88 MHz : dspsigops/Upsample  N=4  phase=0  InputProcessing=Columns as channels (frame based)  RateOptions=Enforce single-rate processing  ic=0  mode=Unused parameter value
  Tx signal : Outport
  Diagnostics : Outport  Port=2
  wires:
  Mix to appropriate hop frequency/1 -> Enabled Subsystem/1(In1)
  Digital Filter Design/1 -> Gain1/1
  Upsample to 88 MHz/1 -> Gain/1
  Gain/1 -> Digital Filter Design/1
  22MHz white noise/1 -> Upsample to 88 MHz/1
  Poisson pulses/1(enable) -> Enabled Subsystem/Enable, Bus Creator/1  "Interf ON"
  M-FSK Modulator Baseband/1 -> Mix to appropriate hop frequency/2
  Constant5/1 -> Sum/1
  Constant1/1 -> Sum/2
  Sum/1 -> Bus Creator/2, M-FSK Modulator Baseband/1  "Interf freq idx"
  Enabled Subsystem/1(Out3) -> Tx signal/1
  Gain1/1 -> Mix to appropriate hop frequency/1
  Bus Creator/1 -> Diagnostics/1

== system BLE_Library/BLE master ==
  Rx signal : Inport
  Constant1 : Constant  SampleTime=Slot_Ts
  Constant4 : Constant  OutDataTypeStr=boolean  SampleTime=Slot_Ts
  Manual Switch1 : ManualSwitch
  Manual Switch4 : ManualSwitch
  Master mode : Subsystem  Variant=on  OverrideUsingVariant=OneSlaveMode
  Rising edge : BLE_Library/Rising edge  SystemSampleTime=-1
  Subsystem7 : Subsystem
      mask Display: disp('Rx\nOn/Off')
  Turn ON time : Delay  DelayLength=tON  InitialCondition=0  SampleTime=Slot_Ts
  Unit Delay1 : UnitDelay  SampleTime=Slot_Ts
  Tx signal : Outport
  Diagnostics : Outport  Port=2
  wires:
  Manual Switch4/1 -> Master mode/3(In3)
  Manual Switch1/1 -> Master mode/2(Rx signal)
  Rising edge/1 -> Master mode/1(Turn ON)
  Master mode/2(Diagnostics) -> Diagnostics/1
  Master mode/1(Tx signal) -> Tx signal/1
  Rx signal/1 -> Unit Delay1/1
  Unit Delay1/1 -> Subsystem7/1(In1), Manual Switch1/1
  Subsystem7/2(Out2) -> Manual Switch4/2
  Constant4/1 -> Manual Switch4/1
  Subsystem7/1(Out1) -> Manual Switch1/2
  Constant1/1 -> Turn ON time/1
  Turn ON time/1 -> Rising edge/1

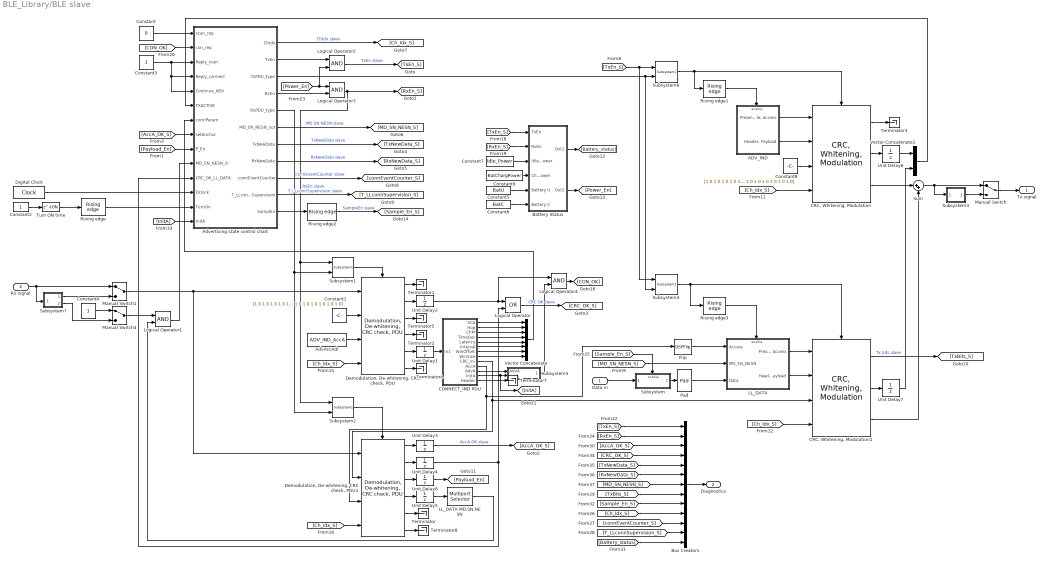
== system BLE_Library/BLE slave ==
  "Data in " : Inport
  Rx signal : Inport  Port=2
  ADV_IND : Subsystem  TreatAsAtomicUnit=on
  AdvAccAdr : Constant  Value=ADV_IND_AccA  VectorParams1D=off  SampleTime=Slot_Ts
  Advertising state control chart : Stateflow chart  TreatAsAtomicUnit=on
  Battery Status : Subsystem
  Bus Creator1 : BusCreator  Inputs=13
  CONNECT_IND PDU : Subsystem
  "CRC, Whitening, Modulation" : BLE_Library/CRC, Whitening,  Modulation
  "CRC, Whitening, Modulation1" : BLE_Library/CRC, Whitening,  Modulation
  Constant : Constant  Value=0  SampleTime=Slot_Ts
  Constant1 : Constant  Value=[1 0 1 0 1 0 1 0 1 0 1 0 1 0 1 0 1 0 1 0 1 0 1 0]  OutDataTypeStr=boolean  SampleTime=Slot_Ts
  Constant2 : Constant  SampleTime=Slot_Ts
  Constant3 : Constant  SampleTime=Slot_Ts
  Constant4 : Constant  OutDataTypeStr=boolean  SampleTime=Slot_Ts
  Constant5 : Constant  Value=BatU  SampleTime=Slot_Ts
  Constant6 : Constant  Value=BatC  SampleTime=Slot_Ts
  Constant7 : Constant  Value=Idle_Power  SampleTime=Slot_Ts
  Constant8 : Constant  Value=[1 0 1 0 1 0 1 0 1 0 1 0 1 0 1 0 1 0 1 0 1 0 1 0]  OutDataTypeStr=boolean  SampleTime=Slot_Ts
  Constant9 : Constant  Value=BatChargPower  SampleTime=Slot_Ts
  "Demodulation, De-whitening, CRC check, PDU" : BLE_Library/Demodulation, De-whitening, CRC check, PDU  PDU_Length=288 %CONNECT_IND: 2+6+6+22 octets (H,InitA,AdvA,LLData)  N_after=312 %max PDU length + CRC
  "Demodulation, De-whitening, CRC check, PDU1" : BLE_Library/Demodulation, De-whitening, CRC check, PDU  PDU_Length=2 %PDU is not required  N_after=40 %max PDU length + CRC
  Digital Clock : DigitalClock  SampleTime=Slot_Ts
  Flip : DSPFlip
  LL_DATA : Subsystem
  LL_DATA MD,SN,NESN : dspindex/Multiport Selector  rowsOrCols=Rows  idxCellArray={12:14}  idxErrMode=Clip Index
  Logical Operator : Logic  Operator=OR  AllPortsSameDT=off  OutDataTypeStr=boolean
  Logical Operator{1..4} (4 alike) : Logic  AllPortsSameDT=off  OutDataTypeStr=boolean
  Manual Switch : ManualSwitch
  Manual Switch1 : ManualSwitch
  Manual Switch4 : ManualSwitch
  Pad : dspsigops/Pad  padAlong=Columns  dimsToPad=1  valSrc=Specify via dialog  padVal=0  spec=Output size  padNumOutRowsSpecMethod=User-specified  numOutRows=n_data*8  padNumOutColsSpecMethod=User-specified  numOutCols=1  isVarDimsMode=off  padBeginning=0  padEnd=0  outSizeMode=User-specified  outSize=1  padSigAt=End  trunc_flag=Warning  roundingMode=Floor  overflowMode=off  truncOrWrapMode=Truncate  wrap_flag=None
      settings: SourceProductName=DSP System Toolbox  SourceProductBaseCode=DS
  Rising edge{,1..3} (4 alike) : BLE_Library/Rising edge  SystemSampleTime=-1
  Subsystem : Subsystem
  Subsystem1 : BLE_Library/Subsystem1  PDU_type=CONNECT_IND_id
  Subsystem2 : BLE_Library/Subsystem1  PDU_type=LL_DATA_id
  Subsystem3 : Subsystem
      mask Display: disp('Tx\nOn/Off')
  Subsystem4 : BLE_Library/Subsystem1  PDU_type=LL_DATA_id
  Subsystem5 : Subsystem
  Subsystem6 : BLE_Library/Subsystem1  PDU_type=ADV_IND_id
  Subsystem7 : Subsystem
      mask Display: disp('Rx\nOn/Off')
  Sum : Sum  Inputs=|++
  Terminator{,1..5,7..8} (8 alike) : Terminator
  Turn ON time : Delay  DelayLength=tON  InitialCondition=0  SampleTime=Slot_Ts
  Unit Delay{1..8} (8 alike) : UnitDelay  SampleTime=Slot_Ts
  Vector Concatenate : Concatenate  NumInputs=8
  Vector Concatenate1 : Concatenate
  Tx signal : Outport
  Diagnostics : Outport  Port=2
  wires:
  Rising edge3/1 -> LL_DATA/Enable
  Subsystem4/1 -> Rising edge3/1, "CRC, Whitening, Modulation1"/Enable
  Rising edge1/1 -> ADV_IND/Enable
  Unit Delay6/1 -> Vector Concatenate1/1
  Subsystem6/1 -> "CRC, Whitening, Modulation"/Enable, Rising edge1/1
  [Sample_En_S] -> Subsystem/Enable
  Rising edge2/1 -> [Sample_En_S]  "SampleEn slave"
  Subsystem/1(Data out) -> Pad/1
  "Data in "/1 -> Subsystem/1(Data in)
  Advertising state control chart/2(TxEn) -> Logical Operator2/1
  Logical Operator3/1 -> [RxEn_S], Subsystem2/1, Subsystem1/1  "RxEn slave"
  Logical Operator2/1 -> [TxEn_S]  "TxEn slave"
  [Power_En] -> Logical Operator2/2, Logical Operator3/1
  "Demodulation, De-whitening, CRC check, PDU1"/2 -> Unit Delay4/1
  "Demodulation, De-whitening, CRC check, PDU1"/1 -> Unit Delay3/1
  "Demodulation, De-whitening, CRC check, PDU"/6 -> Terminator4/1
  "CRC, Whitening, Modulation1"/1 -> [TxBits_S]  "Tx bits slave"
  CONNECT_IND PDU/13(Header) -> Terminator7/1
  CONNECT_IND PDU/12(InitA) -> [InitA], Subsystem5/2(InitA)
  "Demodulation, De-whitening, CRC check, PDU"/4 -> Terminator2/1
  "Demodulation, De-whitening, CRC check, PDU"/1 -> Terminator1/1
  [Ch_Idx_S] -> "Demodulation, De-whitening, CRC check, PDU1"/4
  [Ch_Idx_S] -> "Demodulation, De-whitening, CRC check, PDU"/4
  [Ch_Idx_S] -> "CRC, Whitening, Modulation1"/4
  [Ch_Idx_S] -> "CRC, Whitening, Modulation"/4
  [MD_SN_NESN_S] -> LL_DATA/2(MD_SN_NESN)
  [TxEn_S] -> Subsystem4/1, Subsystem6/1
  [AccA_OK_S] -> Advertising state control chart/8(setAnchor)
  Pad/1 -> LL_DATA/3(Data)
  Advertising state control chart/11(SamplEn) -> Rising edge2/1
  Logical Operator1/1 -> Advertising state control chart/10(MD_SN_NESN_in)
  Manual Switch1/1 -> "Demodulation, De-whitening, CRC check, PDU1"/1, "Demodulation, De-whitening, CRC check, PDU"/1
  Rising edge/1 -> Advertising state control chart/13(TurnOn)
  Turn ON time/1 -> Rising edge/1
  Constant2/1 -> Turn ON time/1
  Digital Clock/1 -> Advertising state control chart/12(Dclock)
  Advertising state control chart/10(T_LLconnSupervision) -> [T_LLconnSupervision_S]  "T_LLconnSupervision slave"
  Advertising state control chart/9(connEventCounter) -> [connEventCounter_S]  "connEventCounter slave"
  Vector Concatenate1/1 -> Advertising state control chart/6(TXACTIVE)
  Unit Delay7/1 -> Vector Concatenate1/2
  "CRC, Whitening, Modulation1"/2 -> Unit Delay7/1
  Advertising state control chart/6(MD_SN_NESN_out) -> [MD_SN_NESN_S]  "MD SN NESN slave"
  Advertising state control chart/8(RxNewData) -> [RxNewData_S]  "RxNewData slave"
  Advertising state control chart/7(TxNewData) -> [TxNewData_S]  "TxNewData slave"
  Unit Delay4/1 -> Advertising state control chart/11(CRC_OK_LL_DATA), Logical Operator/2
  "Demodulation, De-whitening, CRC check, PDU"/2 -> Unit Delay2/1
  "Demodulation, De-whitening, CRC check, PDU"/5 -> Unit Delay1/1
  Unit Delay5/1 -> LL_DATA MD,SN,NESN/1
  LL_DATA MD,SN,NESN/1 -> Logical Operator1/2
  Flip/1 -> LL_DATA/1(Access)
  LL_DATA/2("Header, Payload") -> "CRC, Whitening, Modulation1"/2
  LL_DATA/1("Preamble, Access") -> "CRC, Whitening, Modulation1"/1
  "CRC, Whitening, Modulation1"/3 -> Sum/2
  "CRC, Whitening, Modulation"/3 -> Sum/1
  Advertising state control chart/3(TxPDU_type) -> Subsystem4/2, Subsystem6/2
  Subsystem2/1 -> "Demodulation, De-whitening, CRC check, PDU1"/Enable
  Subsystem1/1 -> "Demodulation, De-whitening, CRC check, PDU"/Enable
  Unit Delay3/1 -> [AccA_OK_S]  "AccA OK slave"
  CONNECT_IND PDU/4(TimeOut) -> Vector Concatenate/4
  CONNECT_IND PDU/5(Latency) -> Vector Concatenate/5
  CONNECT_IND PDU/6(Interval) -> Vector Concatenate/6
  CONNECT_IND PDU/7(WinOffset) -> Vector Concatenate/7
  CONNECT_IND PDU/8(WinSize) -> Vector Concatenate/8
  CONNECT_IND PDU/3(ChM) -> Vector Concatenate/3
  CONNECT_IND PDU/2(Hop) -> Vector Concatenate/2
  CONNECT_IND PDU/1(SCA) -> Vector Concatenate/1
  CONNECT_IND PDU/9(CRC_ini) -> "CRC, Whitening, Modulation1"/3, "Demodulation, De-whitening, CRC check, PDU1"/2
  AdvAccAdr/1 -> "Demodulation, De-whitening, CRC check, PDU"/3
  Logical Operator/1 -> [CRC_OK_S]  "CRC OK slave"
  Unit Delay1/1 -> CONNECT_IND PDU/1(In1)
  Advertising state control chart/5(RxPDU_type) -> Subsystem1/2, Subsystem2/2
  Constant1/1 -> "Demodulation, De-whitening, CRC check, PDU"/2
  Constant8/1 -> "CRC, Whitening, Modulation"/3
  Vector Concatenate/1 -> Advertising state control chart/7(connParam)
  Unit Delay2/1 -> Logical Operator/1, Logical Operator4/1
  Rx signal/1 -> Manual Switch1/1, Subsystem7/1(In1)
  Constant3/1 -> Advertising state control chart/5(Continue_ADV), Advertising state control chart/4(Reply_connect), Advertising state control chart/3(Reply_scan)
  "CRC, Whitening, Modulation"/2 -> Unit Delay6/1
  Constant/1 -> Advertising state control chart/1(scan_req)
  Advertising state control chart/1(ChIdx) -> [Ch_Idx_S]  "ChIdx slave"
  Advertising state control chart/4(RxEn) -> Logical Operator3/2
  ADV_IND/1("Preamble, Access") -> "CRC, Whitening, Modulation"/1
  ADV_IND/2("Header, Payload") -> "CRC, Whitening, Modulation"/2
  Sum/1 -> Subsystem3/1(In1), Manual Switch/1
  [TxEn_S] -> Battery Status/1(TxEn)
  [RxEn_S] -> Battery Status/2(RxEn)
  Constant7/1 -> Battery Status/3(Idle power)
  Battery Status/2(Out2) -> [Power_En]
  Constant5/1 -> Battery Status/5(Battery U)
  Constant6/1 -> Battery Status/6(Battery C)
  Battery Status/1(Out1) -> [Battery_status]
  Manual Switch/1 -> Tx signal/1
  Logical Operator4/1 -> [CON_OK]
  Subsystem5/1(CON OK) -> Logical Operator4/2
  [CON_OK] -> Advertising state control chart/2(con_req)
  CONNECT_IND PDU/10(AccA) -> Flip/1, "Demodulation, De-whitening, CRC check, PDU1"/3
  CONNECT_IND PDU/11(AdvA) -> Subsystem5/1(AdvA)
  [InitA] -> Advertising state control chart/14(InitA)
  Subsystem3/1(Out1) -> Manual Switch/2
  Subsystem7/1(Out1) -> Manual Switch1/2
  Constant4/1 -> Manual Switch4/1
  Subsystem7/2(Out2) -> Manual Switch4/2
  Manual Switch4/1 -> Logical Operator1/1
  [Ch_Idx_S] -> Bus Creator1/10
  [TxNewData_S] -> Bus Creator1/5
  [Sample_En_S] -> Bus Creator1/9
  [AccA_OK_S] -> Bus Creator1/3
  [MD_SN_NESN_S] -> Bus Creator1/7
  [TxEn_S] -> Bus Creator1/1
  [TxBits_S] -> Bus Creator1/8
  Bus Creator1/1 -> Diagnostics/1
  [CRC_OK_S] -> Bus Creator1/4
  [T_LLconnSupervision_S] -> Bus Creator1/12
  [Battery_status] -> Bus Creator1/13
  [RxNewData_S] -> Bus Creator1/6
  [connEventCounter_S] -> Bus Creator1/11
  [RxEn_S] -> Bus Creator1/2
  Constant9/1 -> Battery Status/4(Charging power)
  "CRC, Whitening, Modulation"/1 -> Terminator3/1
  "Demodulation, De-whitening, CRC check, PDU1"/6 -> Terminator8/1
  "Demodulation, De-whitening, CRC check, PDU1"/5 -> Terminator/1
  "Demodulation, De-whitening, CRC check, PDU1"/4 -> Unit Delay5/1
  "Demodulation, De-whitening, CRC check, PDU"/3 -> Terminator5/1
  "Demodulation, De-whitening, CRC check, PDU1"/3 -> Unit Delay8/1
  [Payload_En] -> Advertising state control chart/9(P_En)
  Unit Delay8/1 -> [Payload_En]

== system BLE_Library/Bit Error Rate ==
  Tx_S : Inport
  Rx_M : Inport  Port=2
  Compare To Zero1 : simulink/Logic and Bit Operations/Compare To Zero  relop=>  OutDataTypeStr=boolean
  Constant : Constant  SampleTime=Slot_Ts
  Demux : Demux  Outputs=2
  Demux1 : Demux  Outputs=2
  Divide1 : Product  Inputs=*/
  Enabled Subsystem1 : Subsystem  TreatAsAtomicUnit=on
  Falling edge : BLE_Library/Falling edge  SystemSampleTime=-1
  Logical Operator : Logic  Operator=NXOR  AllPortsSameDT=off  OutDataTypeStr=boolean
  Logical Operator1 : Logic  AllPortsSameDT=off  OutDataTypeStr=boolean
  Logical Operator3 : Logic  AllPortsSameDT=off  OutDataTypeStr=boolean
  Subsystem4 : BLE_Library/Subsystem2  offset=0
  Subsystem7 : BLE_Library/Subsystem2  offset=0
  Sum1 : Sum  Inputs=|-+
  Switch : Switch  Criteria=u2 > Threshold
  Terminator : Terminator
  Unit Delay1 : UnitDelay  SampleTime=Slot_Ts
  Vector Concatenate2 : Concatenate  NumInputs=3
  Out1 : Outport
  wires:
  Demux1/1 -> Logical Operator/1
  Demux/1 -> Logical Operator/2
  Unit Delay1/1 -> Demux/1
  Demux1/2 -> Terminator/1
  Logical Operator1/1 -> Subsystem7/1
  Tx_S/1 -> Unit Delay1/1
  Demux/2 -> Subsystem4/1, Falling edge/1, Logical Operator1/2
  Logical Operator/1 -> Logical Operator1/1
  Rx_M/1 -> Demux1/1
  Switch/1 -> Divide1/2
  Constant/1 -> Switch/3
  Compare To Zero1/1 -> Logical Operator3/2
  Vector Concatenate2/1 -> Enabled Subsystem1/1(In1)
  Divide1/1 -> Vector Concatenate2/1
  Subsystem4/1 -> Switch/2, Compare To Zero1/1, Switch/1, Vector Concatenate2/3, Sum1/2
  Falling edge/1 -> Logical Operator3/1
  Subsystem7/1 -> Sum1/1
  Sum1/1 -> Vector Concatenate2/2, Divide1/1
  Logical Operator3/1 -> Enabled Subsystem1/Enable
  Enabled Subsystem1/1(Out1) -> Out1/1
